simulink model "sideslip_loop"  (Simulink 8.0)
settings: Solver=ode45  StartTime=0.0  StopTime=100  RelTol=1e-3
values from neighbouring files (symbols this model uses):
  a_beta1 = -den(2)    [computeGains.m]
  a_beta2 = num(2)    [computeGains.m]
  delta_r_max = 45*pi/180    (= 0.785398163397)    [computeGains.m]
undefined symbols (not defined in the file or in its folder): P
settings Model: Creator=beard  LastModifiedBy=Gary
settings DataIOCC: SignalLoggingSaveFormat=ModelDataLogs
settings DebuggingCC: FcnCallInpInsideContextMsg=UseLocalSettings
settings CodeAppCC: CustomSymbolStrType=$N$R$M_T  InternalIdentifier=Shortened
settings GRTTargetCC: CombineOutputUpdateFcns=off  GRTInterface=on

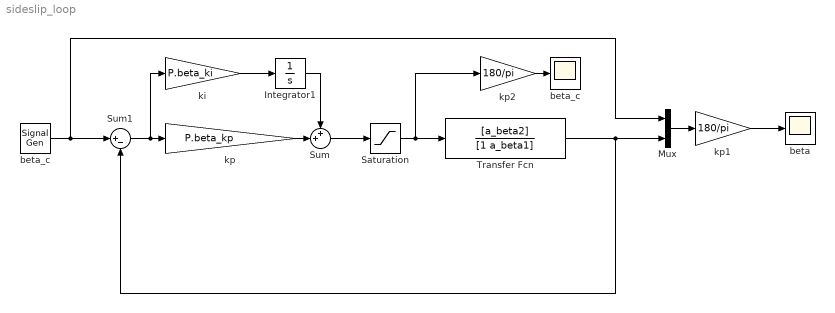
== system sideslip_loop ==
  Integrator1 : Integrator
  Mux : Mux  Inputs=2
  Saturation : Saturate  UpperLimit=delta_r_max  LowerLimit=-delta_r_max
  Sum : Sum  Inputs=++|
  Sum1 : Sum  Inputs=|+-
  Transfer Fcn : TransferFcn  Numerator=[a_beta2]  Denominator=[1 a_beta1]
  beta : Scope
      settings: TimeRange=100  YMin=-100  YMax=100
  beta_c : SignalGenerator  WaveForm=square  Amplitude=25*pi/180  Frequency=.02
  "beta_c " : Scope
      settings: TimeRange=100  YMin=-30  YMax=30
  ki : Gain  Gain=P.beta_ki
  kp : Gain  Gain=P.beta_kp
  kp1 : Gain  Gain=180/pi
  kp2 : Gain  Gain=180/pi
  wires:
  Transfer Fcn/1 -> Sum1/2, Mux/2
  Saturation/1 -> Transfer Fcn/1, kp2/1
  Sum/1 -> Saturation/1
  kp/1 -> Sum/2
  Sum1/1 -> kp/1, ki/1
  ki/1 -> Integrator1/1
  Integrator1/1 -> Sum/1
  beta_c/1 -> Sum1/1, Mux/1
  kp1/1 -> beta/1
  Mux/1 -> kp1/1
  kp2/1 -> "beta_c "/1
